simulink model "ModelOfMotor"  (R2023a)
settings: Solver=VariableStepAuto  StartTime=0.0  StopTime=10.0  RelTol=1e-3
settings Model: Creator=ПК  LastModifiedBy=ПК

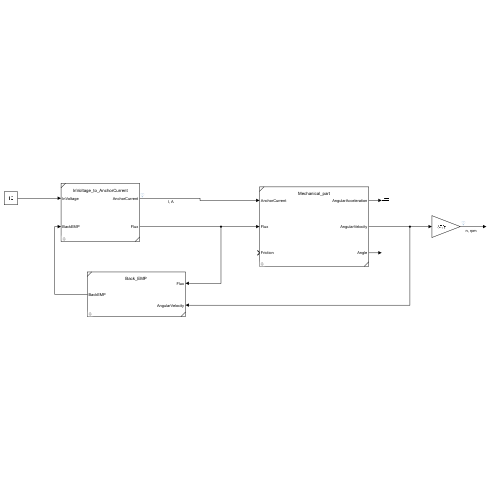
[thumbnail: Simulink's stored preview of the top-level diagram]
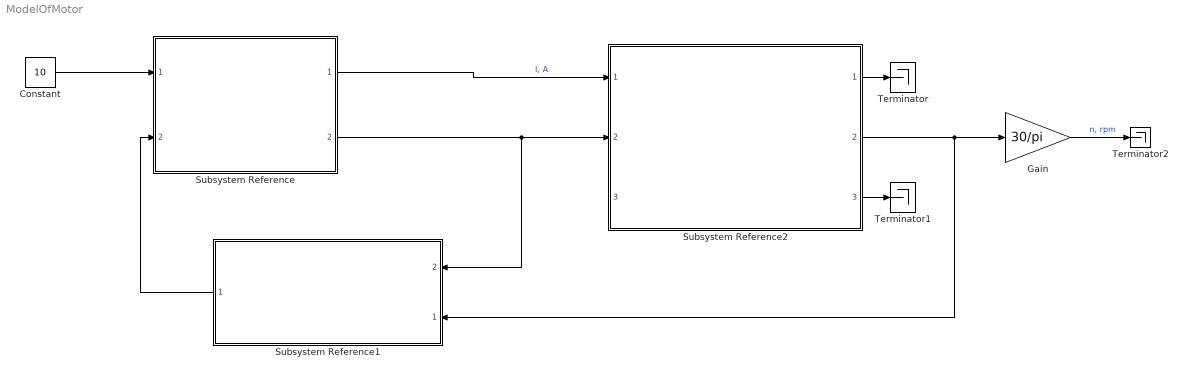
== system ModelOfMotor ==
  Constant : Constant  Value=10
  Gain : Gain  Gain=30/pi
  Subsystem Reference : Subsystem  ReferencedSubsystem=InVoltage_to_AnchorCurrent  R_a=R_a  L_a=L_a  L_ew=L_ew
  Subsystem Reference1 : Subsystem  ReferencedSubsystem=Back_EMP  C_omega=C_omega
      settings: PortSchema="{\"entries\":[{\"content\":{\"sides\":[{\"content\":{\"connectorIds\":[\"In2\",\"In1\"]},\"type\":\"ConnectorPlacement.EquallySpacedRectSide\",\"uuid\":\"3b001cd2-0eb1-4e79-bfc0-23597a26966a\"},{\"content\":{\"connectorIds\":[\"Out1\"],\"side\":\"RIGHT\"},\"type\":\"ConnectorPlacement.EquallySpacedRectSide\",\"uuid\":\"d4852c84-8cb3-4d1c-be31-f1725de136a3\"},{\"content\":{\"side\":\"TOP\"},\"type\":\"ConnectorPlacement.EquallySpacedRectSide\",\"uuid\":\"438efce8-420b-479c-a06d-e294ddb510b6\"}]},\"type\":\"ConnectorPlacement.EquallySpacedConnector\",\"uuid\":\"2b438900-7162-4590-9ac1-dcf2f057e278\"}],\"packageUris\":[\"http://schema.mathworks.com/mf0/Connector/R2020b\"],\"version\":\"1.0\"}"
  Subsystem Reference2 : Subsystem  ReferencedSubsystem=Mechanical_part  C_M=C_M  J_m=J_m
  Terminator : Terminator
  Terminator1 : Terminator
  Terminator2 : Terminator
  wires:
  Constant/1 -> Subsystem Reference/1
  Subsystem Reference/1 -> Subsystem Reference2/1  "I, A"
  Subsystem Reference/2 -> Subsystem Reference2/2, Subsystem Reference1/2
  Subsystem Reference2/2 -> Gain/1, Subsystem Reference1/1
  Subsystem Reference1/1 -> Subsystem Reference/2
  Subsystem Reference2/1 -> Terminator/1
  Subsystem Reference2/3 -> Terminator1/1
  Gain/1 -> Terminator2/1  "n, rpm"
